simulink model "dsp48_macro"  (Simulink 7.6)
settings: Solver=ode45  StartTime=0.0  StopTime=10  RelTol=1e-3
undefined symbols (not defined in the file): xlipgetpartsetting
libraries: xbsIndex_r4 x11, xbsCopyrightNotice_r4 x1
(part 2 of 2)

== system dsp48_macro/More Info ==
